simulink model "DSB_SC"  (R2019a)
settings: Solver=VariableStepAuto  StartTime=0.0  StopTime=inf  RelTol=1e-3
libraries: dsparch4 x1, dspsnks4 x1
settings Model: Creator=Dawson  LastModifiedBy=Dawson
settings SolverCC: AutoInsertRateTranBlk=on
settings DataIOCC: LimitDataPoints=on  SaveOutput=off  SaveTime=off
settings OptimizationCC: BooleanDataType=off  DefaultParameterBehavior=Inlined  LocalBlockOutputs=off  LifeSpan=inf
settings DebuggingCC: AlgebraicLoopMsg=error  SingleTaskRateTransMsg=error  AllowSymbolicDim=off  SFUnexpectedBacktrackingDiag=warning  SFNoUnconditionalDefaultTransitionDiag=warning  SFExecutionAtInitializationDiag=none  ArithmeticOperatorsInVariantConditions=warning
settings SFSimCC: SimUseLocalCustomCode=off
settings RTWCC: RTWUseLocalCustomCode=off
settings CodeAppCC: StateflowObjectComments=on
settings GRTTargetCC: TargetLangStandard=C89/C90 (ANSI)  GeneratePreprocessorConditionals=Disable all
settings ConfigComp: CovMetricSettings=dw  CovHtmlReporting=on  CovSaveCumulativeToWorkspaceVar=on  CovSaveSingleToWorkspaceVar=on  CovExternalEMLEnable=off  CovSFcnEnable=off

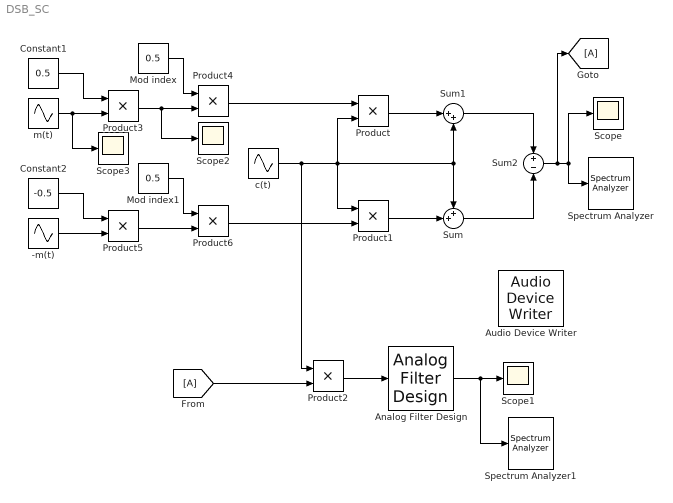
== system DSB_SC ==
  -m(t) : Sin  Amplitude=2  Frequency=2*pi*10  Phase=pi/2  SampleTime=.0005
  Analog Filter Design : dsparch4/Analog Filter Design  method=Butterworth  filttype=Lowpass  N=8  Wlo=2*pi*10  Whi=80  Rp=2  Rs=40
  Audio Device Writer : dspsnks4/Audio Device Writer  Driver=DirectSound  Device=Default  InheritSampleRate=on  SampleRate=44100  BitDepth=16-bit integer  BufferSize=4096  NumBuffers=10  DefaultOutputChannelMapping=on  OutputChannelMapping=1:2  OutputNumUnderrunSamples=off  DriverIdx=1  DeviceWarnFlag=''
  Constant1 : Constant  Value=0.5
  Constant2 : Constant  Value=-0.5
  Mod index : Constant  Value=0.5
  Mod index1 : Constant  Value=0.5
  Product{,1..6} (7 alike) : Product
  Scope{,1..3} (4 alike) : Scope
  Spectrum Analyzer : SpectrumAnalyzer
  Spectrum Analyzer1 : SpectrumAnalyzer
  Sum : Sum  Inputs=++|
  Sum1 : Sum  Inputs=|++
  Sum2 : Sum  Inputs=+|-
  c(t) : Sin  Amplitude=2  Frequency=2*pi*100  Phase=pi/2  SampleTime=.0005
  "m(t) " : Sin  Amplitude=2  Frequency=2*pi*10  Phase=pi/2  SampleTime=.0005
  wires:
  Constant1/1 -> Product3/1
  "m(t) "/1 -> Scope3/1, Product3/2
  Product3/1 -> Scope2/1, Product4/2
  Mod index/1 -> Product4/1
  Product5/1 -> Product6/2
  Mod index1/1 -> Product6/1
  -m(t)/1 -> Product5/2
  Constant2/1 -> Product5/1
  Product6/1 -> Product1/2
  Product4/1 -> Product/1
  c(t)/1 -> Product2/1, Sum1/2, Sum/1, Product/2, Product1/1
  Product/1 -> Sum1/1
  Product1/1 -> Sum/2
  Sum1/1 -> Sum2/1
  Sum/1 -> Sum2/2
  Sum2/1 -> [A], Scope/1, Spectrum Analyzer/1
  [A] -> Product2/2
  Product2/1 -> Analog Filter Design/1
  Analog Filter Design/1 -> Spectrum Analyzer1/1, Scope1/1
